simulink model "Enc"  (R2022b)
settings: Solver=FixedStepDiscrete  StartTime=0.0  StopTime=10.0  FixedStep=0.1  RelTol=1e-3
undefined symbols (not defined in the file): ParamCfg_Avgcnt_u16, ParamCfg_Cosamp_u16, ParamCfg_Cosavg_u16, ParamCfg_Sinamp_u16, ParamCfg_Sinavg_u16
libraries: simulink x2, dspsrcs4 x1
settings Model: DataDictionary=MCU_Input_Sldd.sldd  Creator=ZYH  LastModifiedBy=ZYH
settings OptimizationCC: DefaultParameterBehavior=Inlined  DefaultUnderspecifiedDataType=single  EnhancedBackFolding=on  PassReuseOutputArgsAs=Individual arguments  ZeroExternalMemoryAtStartup=off  ZeroInternalMemoryAtStartup=off  OptimizeBlockOrder=speed  DifferentSizesBufferReuse=on  OptimizationCustomize=off  EfficientTunableParamExpr=on
settings DebuggingCC: ParameterTunabilityLossMsg=error
settings SFSimCC: MATLABDynamicMemAlloc=off
settings RTWCC: Description=Embedded Coder  SystemTargetFile=ert.tlc  GenCodeOnly=on  TemplateMakefile=ert_default_tmf
settings CodeAppCC: IgnoreCustomStorageClasses=off  MaxIdLength=40  OperatorAnnotations=on  SimulinkDataObjDesc=on  SFDataObjDesc=on  SimulinkBlockComments=off
settings ERTTargetCC: TargetLangStandard=C99 (ISO)  GenerateSampleERTMain=on  InlinedParameterPlacement=NonHierarchical  ERTCustomFileTemplate=example_file_process.tlc

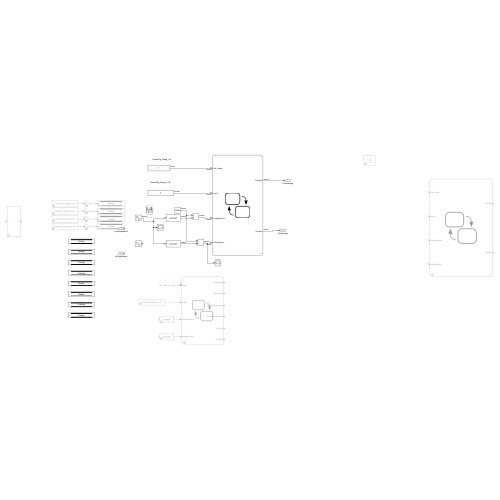
[thumbnail: Simulink's stored preview of the top-level diagram]
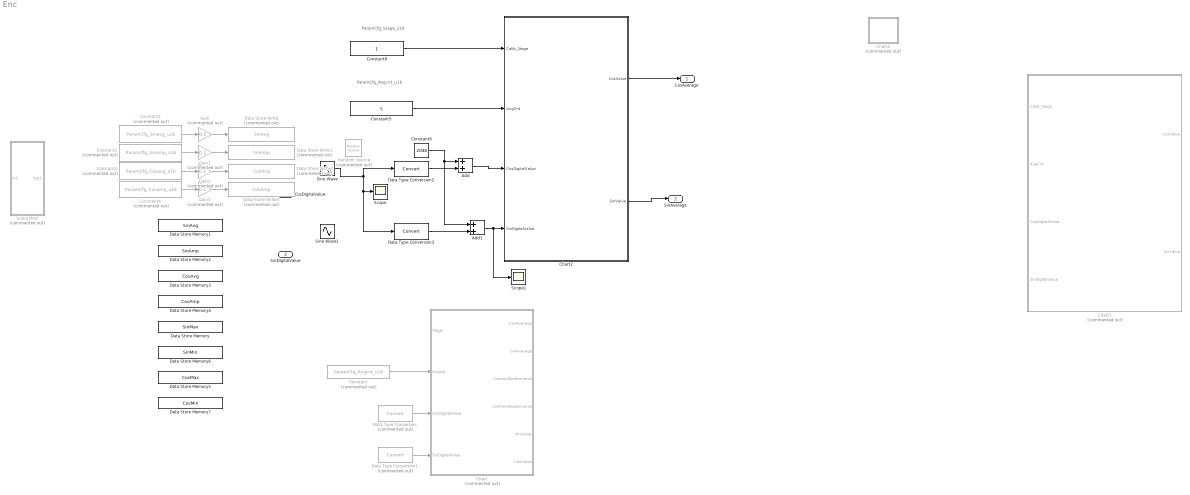
== system Enc ==
  note: ParamCfg_Stage_u16
  note: ParamCfg_Avgcnt_u16
  CosDigitalValue : Inport
  SinDigitalValue : Inport  Port=2
  Add : Sum
  Add1 : Sum
  Chart : Stateflow chart  Commented=on  TreatAsAtomicUnit=on
  Chart1 : Stateflow chart  Commented=on  TreatAsAtomicUnit=on
  Chart2 : Stateflow chart  TreatAsAtomicUnit=on
  Chart3 : Stateflow chart  Commented=on  TreatAsAtomicUnit=on
  Constant : Constant  Commented=on  Value=ParamCfg_Avgcnt_u16
  Constant1 : Constant  Commented=on  Value=ParamCfg_Sinavg_u16
  Constant2 : Constant  Commented=on  Value=ParamCfg_Sinamp_u16
  Constant3 : Constant  Commented=on  Value=ParamCfg_Cosavg_u16
  Constant4 : Constant  Commented=on  Value=ParamCfg_Cosamp_u16
  Constant5 : Constant  Value=5
  Constant6 : Constant  Value=2048
  Constant8 : Constant  OutDataTypeStr=uint16
  Data Store Memory : DataStoreMemory  DataStoreName=SinMax  WriteAfterWriteMsg=warning  InitialValue=2048  ShowAdditionalParam=off
  Data Store Memory1 : DataStoreMemory  DataStoreName=SinAvg  WriteAfterWriteMsg=warning  InitialValue=ParamCfg_Sinavg_u16  ShowAdditionalParam=off  OutDataTypeStr=uint16  StateMustResolveToSignalObject=on
  Data Store Memory2 : DataStoreMemory  DataStoreName=SinAmp  WriteAfterWriteMsg=warning  InitialValue=ParamCfg_Sinamp_u16  ShowAdditionalParam=off  OutDataTypeStr=uint16
  Data Store Memory3 : DataStoreMemory  DataStoreName=CosAvg  WriteAfterWriteMsg=warning  InitialValue=ParamCfg_Cosavg_u16  ShowAdditionalParam=off  OutDataTypeStr=uint16  StateMustResolveToSignalObject=on
  Data Store Memory4 : DataStoreMemory  DataStoreName=CosAmp  WriteAfterWriteMsg=warning  InitialValue=ParamCfg_Cosamp_u16  ShowAdditionalParam=off  OutDataTypeStr=uint16
  Data Store Memory5 : DataStoreMemory  DataStoreName=CosMax  WriteAfterWriteMsg=warning  InitialValue=2048  ShowAdditionalParam=off
  Data Store Memory6 : DataStoreMemory  DataStoreName=SinMin  WriteAfterWriteMsg=warning  InitialValue=2048  ShowAdditionalParam=off
  Data Store Memory7 : DataStoreMemory  DataStoreName=CosMin  WriteAfterWriteMsg=warning  InitialValue=2048  ShowAdditionalParam=off
  Data Store Write : DataStoreWrite  Commented=on  DataStoreName=SinAvg  IndexOptions=Index vector (dialog)  Indices=1  OutputSizes=1
  Data Store Write1 : DataStoreWrite  Commented=on  DataStoreName=SinAmp  IndexOptions=Index vector (dialog)  Indices=1  OutputSizes=1
  Data Store Write2 : DataStoreWrite  Commented=on  DataStoreName=CosAvg  IndexOptions=Index vector (dialog)  Indices=1  OutputSizes=1
  Data Store Write3 : DataStoreWrite  Commented=on  DataStoreName=CosAmp  IndexOptions=Index vector (dialog)  Indices=1  OutputSizes=1
  Data Type Conversion : DataTypeConversion  Commented=on  SaturateOnIntegerOverflow=off  RndMeth=Floor
  Data Type Conversion1 : DataTypeConversion  Commented=on  SaturateOnIntegerOverflow=off  RndMeth=Floor
  Data Type Conversion2 : DataTypeConversion  SaturateOnIntegerOverflow=off  RndMeth=Floor
  Data Type Conversion3 : DataTypeConversion  SaturateOnIntegerOverflow=off  RndMeth=Floor
  Gain{,1..3} (4 alike) : Gain  Commented=on  Gain=0.1  ParamDataTypeStr=single  OutDataTypeStr=single
  Random Source : dspsrcs4/Random Source  Commented=on  SrcType=Uniform  NormMethod=Ziggurat  CltLength=12  MinVal=1  MaxVal=10  MeanVal=0  VarVal=1  RepMode=Not repeatable  rawSeed=1  IsInherit=off  SampMode=Discrete  SampTime=1  SampFrame=1  DataType=Double  OutComplex=Real  OutputFrames=off
  Scope : Scope
  Scope1 : Scope
  Sine Wave : Sin  Amplitude=2  Phase=pi/2  SampleTime=0
  Sine Wave1 : Sin  Amplitude=0  SampleTime=0
  Subsystem : Subsystem  Commented=on
  CosAverage : Outport
  SinAverage : Outport  Port=2
  wires:
  ? -> Chart/1(Stage)
  Constant/1 -> Chart/2(Avgcnt)
  Data Type Conversion/1 -> Chart/3(CosDigitalValue)
  Data Type Conversion1/1 -> Chart/4(SinDigitalValue)
  Constant1/1 -> Gain/1
  Constant2/1 -> Gain1/1
  Gain/1 -> Data Store Write/1
  Gain1/1 -> Data Store Write1/1
  Constant3/1 -> Gain2/1
  Constant4/1 -> Gain3/1
  Gain2/1 -> Data Store Write2/1
  Gain3/1 -> Data Store Write3/1
  Sine Wave/1 -> Data Type Conversion2/1, Data Type Conversion3/1, Scope/1
  Chart2/1(CosValue) -> CosAverage/1
  Chart2/2(SinValue) -> SinAverage/1
  Constant8/1 -> Chart2/1(Calib_Stage)
  Constant5/1 -> Chart2/2(AvgCnt)
  Data Type Conversion2/1 -> Add/2
  Data Type Conversion3/1 -> Add1/2
  Add1/1 -> Scope1/1, Chart2/4(SinDigitalValue)
  Constant6/1 -> Add1/1, Add/1
  Add/1 -> Chart2/3(CosDigitalValue)

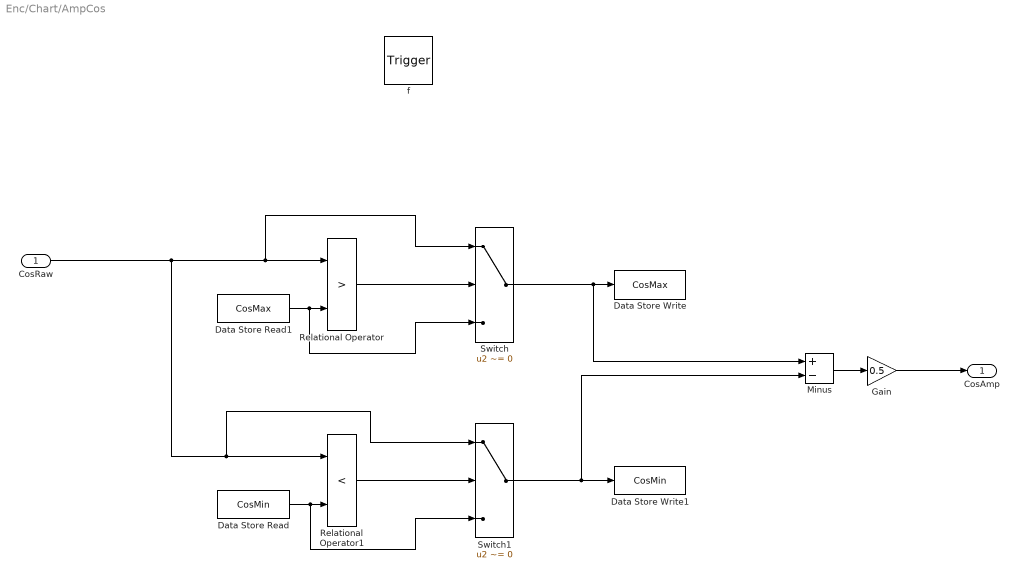
== system Enc/Chart/AmpCos ==
  CosRaw : Inport
  f : TriggerPort  TriggerType=function-call  VariantControl=(inherit)
      settings: CopyFcn=Stateflow.SLINSF.SimulinkMan.removeBlockPreDeleteFcn  PreDeleteFcn=Stateflow.SLINSF.SimulinkMan.unsafePredeleteFcn
  Data Store Read : DataStoreRead  DataStoreName=CosMin  IndexOptions=Index vector (dialog)  Indices=1  OutputSizes=1
  Data Store Read1 : DataStoreRead  DataStoreName=CosMax  IndexOptions=Index vector (dialog)  Indices=1  OutputSizes=1
  Data Store Write : DataStoreWrite  DataStoreName=CosMax  IndexOptions=Index vector (dialog)  Indices=1  OutputSizes=1
  Data Store Write1 : DataStoreWrite  DataStoreName=CosMin  IndexOptions=Index vector (dialog)  Indices=1  OutputSizes=1
  Gain : Gain  Gain=0.5
  Minus : Sum  Inputs=+-
  Relational Operator : RelationalOperator  Operator=>  OutDataTypeStr=boolean  RndMeth=Simplest  InputSameDT=off
  Relational Operator1 : RelationalOperator  Operator=<  OutDataTypeStr=boolean  RndMeth=Simplest  InputSameDT=off
  Switch : Switch  Criteria=u2 ~= 0  SaturateOnIntegerOverflow=off  InputSameDT=off
  Switch1 : Switch  Criteria=u2 ~= 0  SaturateOnIntegerOverflow=off  InputSameDT=off
  CosAmp : Outport
  wires:
  CosRaw/1 -> Switch1/1, Relational Operator1/1, Switch/1, Relational Operator/1
  Data Store Read1/1 -> Switch/3, Relational Operator/2
  Relational Operator/1 -> Switch/2
  Switch/1 -> Minus/1, Data Store Write/1
  Data Store Read/1 -> Switch1/3, Relational Operator1/2
  Relational Operator1/1 -> Switch1/2
  Switch1/1 -> Minus/2, Data Store Write1/1
  Minus/1 -> Gain/1
  Gain/1 -> CosAmp/1

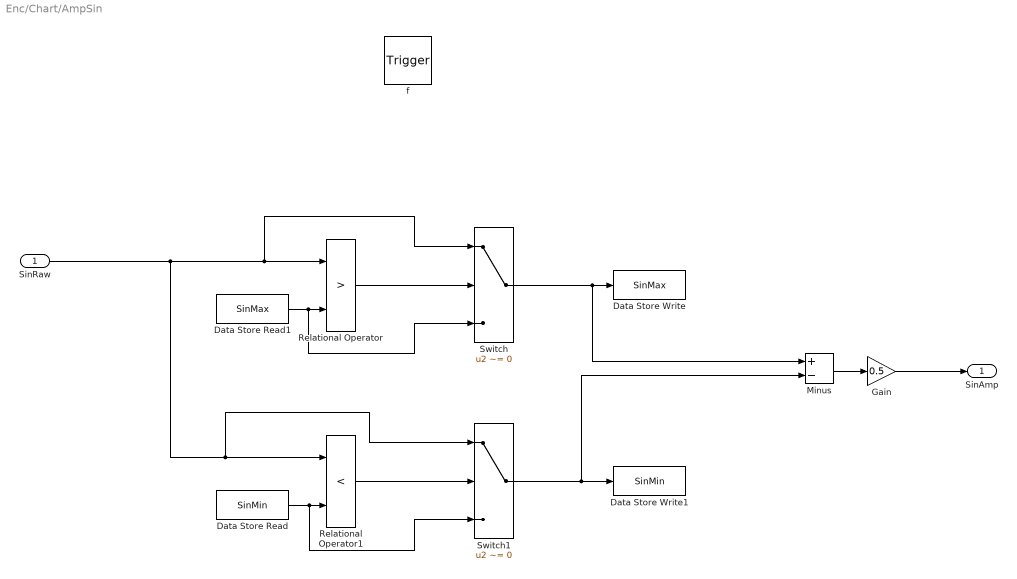
== system Enc/Chart/AmpSin ==
  SinRaw : Inport
  f : TriggerPort  TriggerType=function-call  VariantControl=(inherit)
      settings: CopyFcn=Stateflow.SLINSF.SimulinkMan.removeBlockPreDeleteFcn  PreDeleteFcn=Stateflow.SLINSF.SimulinkMan.unsafePredeleteFcn
  Data Store Read : DataStoreRead  DataStoreName=SinMin  IndexOptions=Index vector (dialog)  Indices=1  OutputSizes=1
  Data Store Read1 : DataStoreRead  DataStoreName=SinMax  IndexOptions=Index vector (dialog)  Indices=1  OutputSizes=1
  Data Store Write : DataStoreWrite  DataStoreName=SinMax  IndexOptions=Index vector (dialog)  Indices=1  OutputSizes=1
  Data Store Write1 : DataStoreWrite  DataStoreName=SinMin  IndexOptions=Index vector (dialog)  Indices=1  OutputSizes=1
  Gain : Gain  Gain=0.5
  Minus : Sum  Inputs=+-
  Relational Operator : RelationalOperator  Operator=>  OutDataTypeStr=boolean  RndMeth=Simplest  InputSameDT=off
  Relational Operator1 : RelationalOperator  Operator=<  OutDataTypeStr=boolean  RndMeth=Simplest  InputSameDT=off
  Switch : Switch  Criteria=u2 ~= 0  SaturateOnIntegerOverflow=off  InputSameDT=off
  Switch1 : Switch  Criteria=u2 ~= 0  SaturateOnIntegerOverflow=off  InputSameDT=off
  SinAmp : Outport
  wires:
  SinRaw/1 -> Switch1/1, Relational Operator1/1, Switch/1, Relational Operator/1
  Data Store Read1/1 -> Switch/3, Relational Operator/2
  Relational Operator/1 -> Switch/2
  Switch/1 -> Minus/1, Data Store Write/1
  Data Store Read/1 -> Switch1/3, Relational Operator1/2
  Relational Operator1/1 -> Switch1/2
  Switch1/1 -> Minus/2, Data Store Write1/1
  Minus/1 -> Gain/1
  Gain/1 -> SinAmp/1

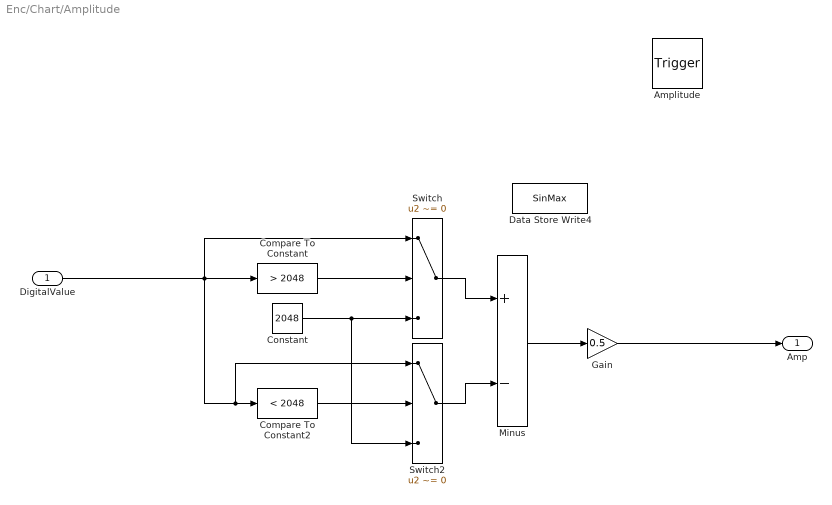
== system Enc/Chart/Amplitude ==
  DigitalValue : Inport  OutMin=0  OutMax=65535  OutDataTypeStr=uint16  PortDimensions=1
  Amplitude : TriggerPort  TriggerType=function-call  VariantControl=(inherit)
      settings: CopyFcn=Stateflow.SLINSF.SimulinkMan.removeBlockPreDeleteFcn  PreDeleteFcn=Stateflow.SLINSF.SimulinkMan.unsafePredeleteFcn
  Compare To Constant : simulink/Logic and Bit Operations/Compare To Constant  relop=>  const=2048  OutDataTypeStr=boolean
  Compare To Constant2 : simulink/Logic and Bit Operations/Compare To Constant  relop=<  const=2048  OutDataTypeStr=boolean
  Constant : Constant  Value=2048  OutDataTypeStr=uint16
  Data Store Write4 : DataStoreWrite  DataStoreName=SinMax  IndexOptions=Index vector (dialog)  Indices=1  OutputSizes=1
  Gain : Gain  Gain=0.5  OutDataTypeStr=single
  Minus : Sum  Inputs=+-
  Switch : Switch  Criteria=u2 ~= 0  SaturateOnIntegerOverflow=off  InputSameDT=off
  Switch2 : Switch  Criteria=u2 ~= 0  SaturateOnIntegerOverflow=off  InputSameDT=off
  Amp : Outport  PortDimensions=1
  wires:
  Compare To Constant/1 -> Switch/2
  Gain/1 -> Amp/1
  Compare To Constant2/1 -> Switch2/2
  Switch/1 -> Minus/1
  Switch2/1 -> Minus/2
  Constant/1 -> Switch2/3, Switch/3
  DigitalValue/1 -> Switch2/1, Compare To Constant2/1, Switch/1, Compare To Constant/1
  Minus/1 -> Gain/1

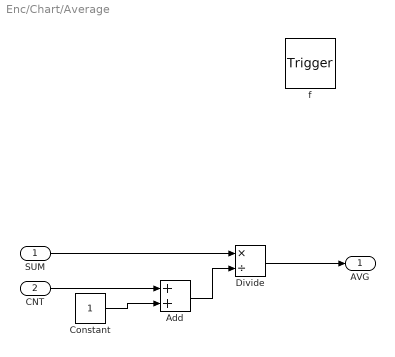
== system Enc/Chart/Average ==
  SUM : Inport  OutDataTypeStr=uint32  PortDimensions=1
  CNT : Inport  Port=2  OutDataTypeStr=uint16  PortDimensions=1
  f : TriggerPort  TriggerType=function-call  VariantControl=(inherit)
      settings: CopyFcn=Stateflow.SLINSF.SimulinkMan.removeBlockPreDeleteFcn  PreDeleteFcn=Stateflow.SLINSF.SimulinkMan.unsafePredeleteFcn
  Add : Sum  OutDataTypeStr=uint16
  Constant : Constant  OutDataTypeStr=uint16
  Divide : Product  Inputs=*/  OutDataTypeStr=single
  AVG : Outport  PortDimensions=1
  wires:
  CNT/1 -> Add/1
  Constant/1 -> Add/2
  SUM/1 -> Divide/1
  Add/1 -> Divide/2
  Divide/1 -> AVG/1

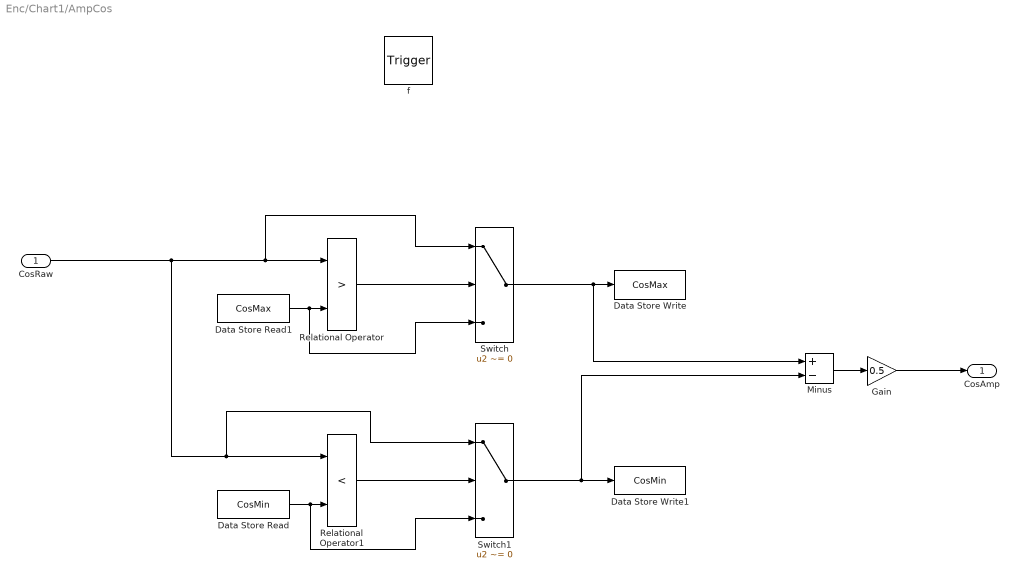
== system Enc/Chart1/AmpCos ==
  CosRaw : Inport  OutDataTypeStr=uint16  PortDimensions=1
  f : TriggerPort  TriggerType=function-call  VariantControl=(inherit)
      settings: CopyFcn=Stateflow.SLINSF.SimulinkMan.removeBlockPreDeleteFcn  PreDeleteFcn=Stateflow.SLINSF.SimulinkMan.unsafePredeleteFcn
  Data Store Read : DataStoreRead  DataStoreName=CosMin  IndexOptions=Index vector (dialog)  Indices=1  OutputSizes=1
  Data Store Read1 : DataStoreRead  DataStoreName=CosMax  IndexOptions=Index vector (dialog)  Indices=1  OutputSizes=1
  Data Store Write : DataStoreWrite  DataStoreName=CosMax  IndexOptions=Index vector (dialog)  Indices=1  OutputSizes=1
  Data Store Write1 : DataStoreWrite  DataStoreName=CosMin  IndexOptions=Index vector (dialog)  Indices=1  OutputSizes=1
  Gain : Gain  Gain=0.5  ParamDataTypeStr=single  OutDataTypeStr=single
  Minus : Sum  Inputs=+-
  Relational Operator : RelationalOperator  Operator=>  OutDataTypeStr=boolean  RndMeth=Simplest  InputSameDT=off
  Relational Operator1 : RelationalOperator  Operator=<  OutDataTypeStr=boolean  RndMeth=Simplest  InputSameDT=off
  Switch : Switch  Criteria=u2 ~= 0  SaturateOnIntegerOverflow=off  InputSameDT=off
  Switch1 : Switch  Criteria=u2 ~= 0  SaturateOnIntegerOverflow=off  InputSameDT=off
  CosAmp : Outport  OutDataTypeStr=single
  wires:
  CosRaw/1 -> Switch1/1, Relational Operator1/1, Switch/1, Relational Operator/1
  Data Store Read1/1 -> Switch/3, Relational Operator/2
  Relational Operator/1 -> Switch/2
  Switch/1 -> Minus/1, Data Store Write/1
  Data Store Read/1 -> Switch1/3, Relational Operator1/2
  Relational Operator1/1 -> Switch1/2
  Switch1/1 -> Minus/2, Data Store Write1/1
  Minus/1 -> Gain/1
  Gain/1 -> CosAmp/1

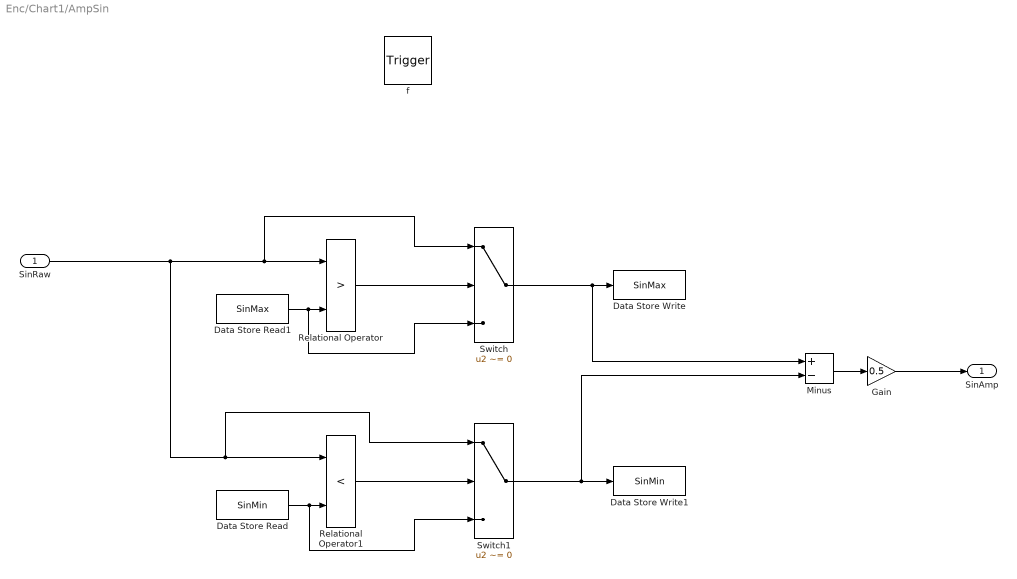
== system Enc/Chart1/AmpSin ==
  SinRaw : Inport  OutDataTypeStr=uint16  PortDimensions=1
  f : TriggerPort  TriggerType=function-call  VariantControl=(inherit)
      settings: CopyFcn=Stateflow.SLINSF.SimulinkMan.removeBlockPreDeleteFcn  PreDeleteFcn=Stateflow.SLINSF.SimulinkMan.unsafePredeleteFcn
  Data Store Read : DataStoreRead  DataStoreName=SinMin  IndexOptions=Index vector (dialog)  Indices=1  OutputSizes=1
  Data Store Read1 : DataStoreRead  DataStoreName=SinMax  IndexOptions=Index vector (dialog)  Indices=1  OutputSizes=1
  Data Store Write : DataStoreWrite  DataStoreName=SinMax  IndexOptions=Index vector (dialog)  Indices=1  OutputSizes=1
  Data Store Write1 : DataStoreWrite  DataStoreName=SinMin  IndexOptions=Index vector (dialog)  Indices=1  OutputSizes=1
  Gain : Gain  Gain=0.5  ParamDataTypeStr=single  OutDataTypeStr=single
  Minus : Sum  Inputs=+-
  Relational Operator : RelationalOperator  Operator=>  OutDataTypeStr=boolean  RndMeth=Simplest  InputSameDT=off
  Relational Operator1 : RelationalOperator  Operator=<  OutDataTypeStr=boolean  RndMeth=Simplest  InputSameDT=off
  Switch : Switch  Criteria=u2 ~= 0  SaturateOnIntegerOverflow=off  InputSameDT=off
  Switch1 : Switch  Criteria=u2 ~= 0  SaturateOnIntegerOverflow=off  InputSameDT=off
  SinAmp : Outport  OutDataTypeStr=single  PortDimensions=1
  wires:
  SinRaw/1 -> Switch1/1, Relational Operator1/1, Switch/1, Relational Operator/1
  Data Store Read1/1 -> Switch/3, Relational Operator/2
  Relational Operator/1 -> Switch/2
  Switch/1 -> Minus/1, Data Store Write/1
  Data Store Read/1 -> Switch1/3, Relational Operator1/2
  Relational Operator1/1 -> Switch1/2
  Switch1/1 -> Minus/2, Data Store Write1/1
  Minus/1 -> Gain/1
  Gain/1 -> SinAmp/1

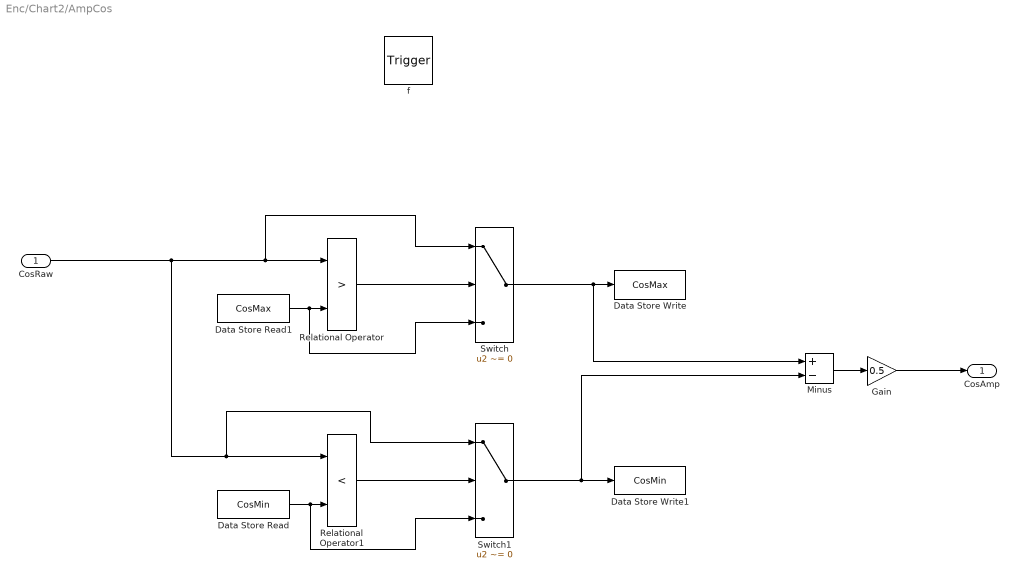
== system Enc/Chart2/AmpCos ==
  CosRaw : Inport  OutDataTypeStr=uint16  PortDimensions=1
  f : TriggerPort  TriggerType=function-call  VariantControl=(inherit)
      settings: CopyFcn=Stateflow.SLINSF.SimulinkMan.removeBlockPreDeleteFcn  PreDeleteFcn=Stateflow.SLINSF.SimulinkMan.unsafePredeleteFcn
  Data Store Read : DataStoreRead  DataStoreName=CosMin  IndexOptions=Index vector (dialog)  Indices=1  OutputSizes=1
  Data Store Read1 : DataStoreRead  DataStoreName=CosMax  IndexOptions=Index vector (dialog)  Indices=1  OutputSizes=1
  Data Store Write : DataStoreWrite  DataStoreName=CosMax  IndexOptions=Index vector (dialog)  Indices=1  OutputSizes=1
  Data Store Write1 : DataStoreWrite  DataStoreName=CosMin  IndexOptions=Index vector (dialog)  Indices=1  OutputSizes=1
  Gain : Gain  Gain=0.5  ParamDataTypeStr=single  OutDataTypeStr=single
  Minus : Sum  Inputs=+-
  Relational Operator : RelationalOperator  Operator=>  OutDataTypeStr=boolean  RndMeth=Simplest  InputSameDT=off
  Relational Operator1 : RelationalOperator  Operator=<  OutDataTypeStr=boolean  RndMeth=Simplest  InputSameDT=off
  Switch : Switch  Criteria=u2 ~= 0  SaturateOnIntegerOverflow=off  InputSameDT=off
  Switch1 : Switch  Criteria=u2 ~= 0  SaturateOnIntegerOverflow=off  InputSameDT=off
  CosAmp : Outport  OutDataTypeStr=single
  wires:
  CosRaw/1 -> Switch1/1, Relational Operator1/1, Switch/1, Relational Operator/1
  Data Store Read1/1 -> Switch/3, Relational Operator/2
  Relational Operator/1 -> Switch/2
  Switch/1 -> Minus/1, Data Store Write/1
  Data Store Read/1 -> Switch1/3, Relational Operator1/2
  Relational Operator1/1 -> Switch1/2
  Switch1/1 -> Minus/2, Data Store Write1/1
  Minus/1 -> Gain/1
  Gain/1 -> CosAmp/1

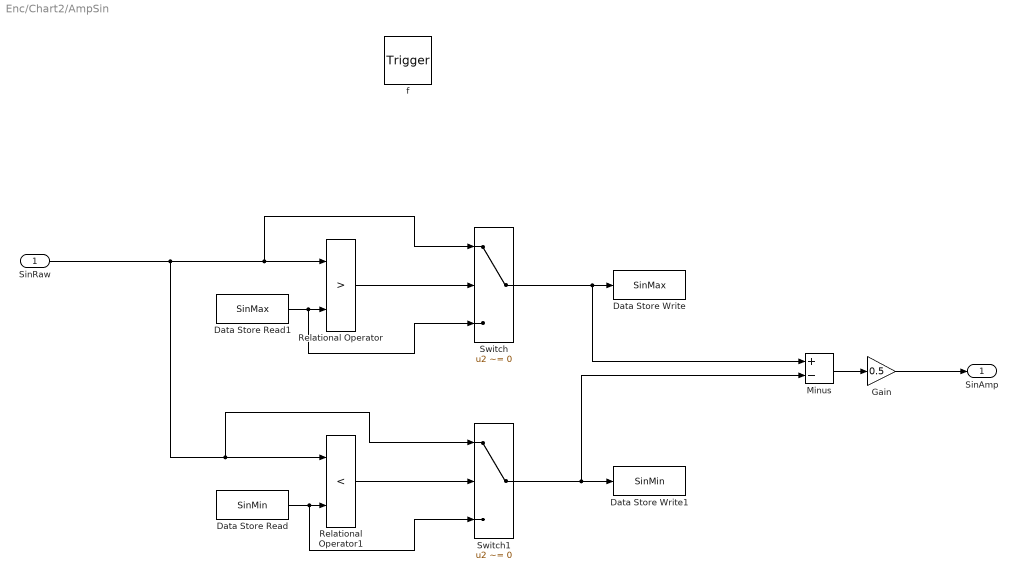
== system Enc/Chart2/AmpSin ==
  SinRaw : Inport  OutDataTypeStr=uint16  PortDimensions=1
  f : TriggerPort  TriggerType=function-call  VariantControl=(inherit)
      settings: CopyFcn=Stateflow.SLINSF.SimulinkMan.removeBlockPreDeleteFcn  PreDeleteFcn=Stateflow.SLINSF.SimulinkMan.unsafePredeleteFcn
  Data Store Read : DataStoreRead  DataStoreName=SinMin  IndexOptions=Index vector (dialog)  Indices=1  OutputSizes=1
  Data Store Read1 : DataStoreRead  DataStoreName=SinMax  IndexOptions=Index vector (dialog)  Indices=1  OutputSizes=1
  Data Store Write : DataStoreWrite  DataStoreName=SinMax  IndexOptions=Index vector (dialog)  Indices=1  OutputSizes=1
  Data Store Write1 : DataStoreWrite  DataStoreName=SinMin  IndexOptions=Index vector (dialog)  Indices=1  OutputSizes=1
  Gain : Gain  Gain=0.5  ParamDataTypeStr=single  OutDataTypeStr=single
  Minus : Sum  Inputs=+-
  Relational Operator : RelationalOperator  Operator=>  OutDataTypeStr=boolean  RndMeth=Simplest  InputSameDT=off
  Relational Operator1 : RelationalOperator  Operator=<  OutDataTypeStr=boolean  RndMeth=Simplest  InputSameDT=off
  Switch : Switch  Criteria=u2 ~= 0  SaturateOnIntegerOverflow=off  InputSameDT=off
  Switch1 : Switch  Criteria=u2 ~= 0  SaturateOnIntegerOverflow=off  InputSameDT=off
  SinAmp : Outport  OutDataTypeStr=single  PortDimensions=1
  wires:
  SinRaw/1 -> Switch1/1, Relational Operator1/1, Switch/1, Relational Operator/1
  Data Store Read1/1 -> Switch/3, Relational Operator/2
  Relational Operator/1 -> Switch/2
  Switch/1 -> Minus/1, Data Store Write/1
  Data Store Read/1 -> Switch1/3, Relational Operator1/2
  Relational Operator1/1 -> Switch1/2
  Switch1/1 -> Minus/2, Data Store Write1/1
  Minus/1 -> Gain/1
  Gain/1 -> SinAmp/1

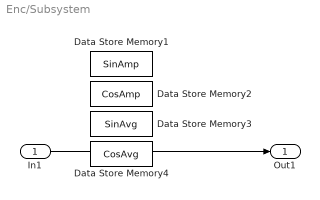
== system Enc/Subsystem ==
  In1 : Inport
  Data Store Memory1 : DataStoreMemory  DataStoreName=SinAmp  WriteAfterWriteMsg=warning  InitialValue=ParamCfg_Sinamp_u16  ShowAdditionalParam=off  OutDataTypeStr=single  StateMustResolveToSignalObject=on
  Data Store Memory2 : DataStoreMemory  DataStoreName=CosAmp  WriteAfterWriteMsg=warning  ShowAdditionalParam=off  OutDataTypeStr=single  StateMustResolveToSignalObject=on
  Data Store Memory3 : DataStoreMemory  DataStoreName=SinAvg  WriteAfterWriteMsg=warning  ShowAdditionalParam=off  OutDataTypeStr=single  StateMustResolveToSignalObject=on
  Data Store Memory4 : DataStoreMemory  DataStoreName=CosAvg  WriteAfterWriteMsg=warning  ShowAdditionalParam=off  OutDataTypeStr=single  StateMustResolveToSignalObject=on
  Out1 : Outport
  wires:
  In1/1 -> Out1/1

== stateflow chart Enc/Chart3 ==
  state A
  (default) -> (junction 3)
  (junction 3) -> A

== stateflow chart Enc/Chart1 ==
  state SinAmp = AmpSin(SinRaw) [function]
  state Normalize
    du:
    if(Cnt < AvgCnt)
    AmplitudeSin =AmpSin(SinDigitalValue);
    AmplitudeCos = AmpCos(CosDigitalValue);
    SinSum = SinSum + SinDigitalValue;
    CosSum = CosSum + CosDigitalValue;
    Cnt = Cnt + 1;
    else
    %求均值
    SinAverage = SinSum/(Cnt+1);
    CosAverage = CosSum/(Cnt+1);
    %求幅值倒数
    InvAmpSin = 1/AmplitudeSin;
    InvAmpCos = 1/AmplitudeCos;
    %更新参数
    end
    end
  state Compensate
  state CosAmp = AmpCos(CosRaw) [function]
  note: NormlizeSinCos
      |
      | du:
      | if(Cnt < Avgcnt)
      |     SinAmplitude = AmpSin(SinDigitalValue);
      |     CosAmplitude = AmpCos(CosDigitalValue);
      |     Cnt = Cnt+1;
      |     SinSum = SinSum + uint32(SinDigitalValue);
      |     CosSum = CosSum+ uint32(CosDigitalValue);
      | else
      |     SinAverage = Average(SinSum,Cnt);%single(SinSum/(Cnt+1));
      |     CosAverage = Average(CosSum,Cnt);%single(CosSum/(Cnt+1));
      |
      |     SinAmplitudeInverse = 1/SinAmplitude;
      |     CosAmplitudeInverse = 1/CosAmplitude;
      |
      |     SinAvg = SinAverage*10;
      |     CosAvg = CosAverage*10;
      |     SinAmp = SinAmplitude*10;
      |     CosAmp = CosAmplitude*10;
      | end
      | ToCalibFinish = true;
      | end
  state Finish
    du:
  (default) -> (junction 7)
  (junction 7) -> Compensate [order 3] : [Calib_Stage == COMPENSATE]
  (junction 7) -> Normalize [order 1] : [Calib_Stage == NORMALIZE]
  (junction 7) -> Finish [order 2]
  Compensate -> Finish
  Normalize -> Finish
  Finish -> (junction 23) : {
      | SinValue =1;
      | CosValue = 1;
      | }
  data: SinRaw function_input uint16 size=1; SinAmp function_output single size=1; CosRaw function_input uint16 size=1; CosAmp function_output single; Calib_Stage input; NORMALIZE constant double; COMPENSATE constant double; CosValue output; SinValue output; AvgCnt input; Cnt local; CosDigitalValue input; SinDigitalValue input; AmplitudeSin local single =single(0); AmplitudeCos local single =single(0); CosSum local s; SinSum local; CosAverage local; SinAverage local; InvAmpCos local; InvAmpSin local

== stateflow chart Enc/Chart2 ==
  note: Normalize
      |
      | du:
      | if(Cnt < AvgCnt)
      |     AmplitudeSin =AmpSin(SinDigitalValue);
      |     AmplitudeCos = AmpCos(CosDigitalValue);
      |     SinSum = SinSum + SinDigitalValue;
      |     CosSum = CosSum + CosDigitalValue;
      |     Cnt = Cnt + 1;
      | else
      |     %求均值
      |     SinAverage = SinSum/(Cnt+1);
      |     CosAverage = CosSum/(Cnt+1);
      |
      |     %求幅值倒数
      |     InvAmpSin = 1/AmplitudeSin;
      |     InvAmpCos = 1/AmplitudeCos;
      |
      |     %更新参数
      |
      | end
      | end
  note: Normalize
      |
      | du:
      | if(Cnt < AvgCnt)
      |     AmplitudeSin =AmpSin(SinDigitalValue);
      |     AmplitudeCos = AmpCos(CosDigitalValue);
      |     SinSum = SinSum + SinDigitalValue;
      |     CosSum = CosSum + CosDigitalValue;
      |     Cnt = Cnt + 1;
      | else
      |     %求均值
      |     SinAverage = SinSum/(Cnt+1);
      |     CosAverage = CosSum/(Cnt+1);
      |
      |     %求幅值倒数
      |     InvAmpSin = 1/AmplitudeSin;
      |     InvAmpCos = 1/AmplitudeCos;
      |
      |     %更新参数
      |
      | end
      | end
  state SinAmp = AmpSin(SinRaw) [function]
  state Normalize
    state A
      SinAmplitude =AmpSin(SinDigitalValue);
      CosAmplitude = AmpCos(CosDigitalValue);
      SinSum = SinSum + SinDigitalValue;
      CosSum = CosSum + CosDigitalValue;
      Cnt = Cnt+1;
    state B
      %求均值
      SinAverage = SinSum/(Cnt);
      CosAverage = CosSum/(Cnt);
      %求幅值倒数
      SinAmplitudeInverse = 1/SinAmplitude;
      CosAmplitudeInverse = 1/CosAmplitude;
      %更新参数
      SinAvg = SinAverage*10;
      CosAvg = CosAverage *10;
      SinAmp = SinAmplitude *10;
      CosAmp = CosAmplitude *10;
      %状态跳转
      ToFinish = 1
    (default) -> A
    (default) -> (junction 42) [commented out]
    (junction 42) -> ? [commented out] : [Cnt <AvgCnt]
        | {
        |     SinAmplitude =AmpSin(SinDigitalValue);
        |     CosAmplitude = AmpCos(CosDigitalValue);
        |     SinSum = SinSum + SinDigitalValue;
        |     CosSum = CosSum + CosDigitalValue;
        |     Cnt = Cnt + 1;
        | }
    (junction 42) -> ? [commented out] : {
        |     %求均值
        |     SinAverage = SinSum/(Cnt+1);
        |     CosAverage = CosSum/(Cnt+1);
        |
        |     %求幅值倒数
        |     SinAmplitudeInverse = 1/SinAmplitude;
        |     CosAmplitudeInverse = 1/CosAmplitude;
        |
        | %更新参数
        | SinAvg = SinAverage*10;
        | CosAvg = CosAverage *10;
        | SinAmp = SinAmplitude *10;
        | CosAmp = CosAmplitude *10;
        |
        | %状态跳转
        | ToFinish = 1
        | }
    A -> B : [Cnt > AvgCnt]
  state Compensate
  state CosAmp = AmpCos(CosRaw) [function]
  state Finish
    SinSum = 0;
    CosSum= 0;
    Cnt = 0;
    SinValue =(SinDigitalValue-SinAvg)*SinAmplitudeInverse;
    CosValue = (CosDigitalValue-CosAvg)*CosAmplitudeInverse;
  (default) -> (junction 7)
  (junction 7) -> Compensate [order 2] : [Calib_Stage == COMPENSATE]
  (junction 7) -> Normalize [order 1] : [Calib_Stage == NORMALIZE]
  (junction 7) -> Finish [order 3]
  Normalize -> Finish : [ToFinish == 1]
  Finish -> (junction 9) [commented out] : {
      | SinValue =(SinDigitalValue-SinAvg)*SinAmplitudeInverse;
      | CosValue = (CosDigitalValue-CosAvg)*CosAmplitudeInverse;
      | }
  data: SinRaw function_input uint16 size=1; SinAmp function_output single size=1; CosRaw function_input uint16 size=1; CosAmp function_output single; Calib_Stage input; AvgCnt input; CosDigitalValue input; SinDigitalValue input; CosValue output double; SinValue output double; Cnt local uint16 =0; CosSum local double; SinSum local double; COMPENSATE constant uint16 =2; NORMALIZE constant uint16 =1; SinAverage local double; CosAverage local double; CosAmplitudeInverse local double; SinAmplitudeInverse local double; CosAmplitude local double; SinAmplitude local double; CosAvg data_store_memory; SinAvg data_store_memory; SinAmp data_store_memory; CosAmp data_store_memory; ToFinish local uint8 =0

== stateflow chart Enc/Chart ==
  state CalibFinish
    du:
    Cnt = 0;
    SinSum = 0;
    CosSum = 0;
    ToCalibFinish = false;
    ToDown = true;
    end
  state SinAmp = AmpSin(SinRaw) [function]
  state IDLE
  state CosAmp = AmpCos(CosRaw) [function]
  state Amp = Amplitude(DigitalValue) [function] [commented out]
  state AVG = Average(SUM,CNT) [function] [commented out]
  state NormlizeSinCos
    du:
    if(Cnt < Avgcnt)
    SinAmplitude = AmpSin(SinDigitalValue);
    CosAmplitude = AmpCos(CosDigitalValue);
    Cnt = Cnt+1;
    SinSum = SinSum + uint32(SinDigitalValue);
    CosSum = CosSum+ uint32(CosDigitalValue);
    else
    SinAverage = Average(SinSum,Cnt);%single(SinSum/(Cnt+1));
    CosAverage = Average(CosSum,Cnt);%single(CosSum/(Cnt+1));
    SinAmplitudeInverse = 1/SinAmplitude;
    CosAmplitudeInverse = 1/CosAmplitude;
    SinAvg = SinAverage*10;
    CosAvg = CosAverage*10;
    SinAmp = SinAmplitude*10;
    CosAmp = CosAmplitude*10;
    end
    ToCalibFinish = true;
    end
  state CompPhaseShift
    SinSum = 1;
    CosSum = 1;
  state Down [commented out]
    du:
    SinValue = (single(SinDigitalValue)-SinAverage) *SinAmplitudeInverse;
    CosValue = (single(CosDigitalValue)-CosAverage)*CosAmplitudeInverse;
  state Up
    du:
    SinValue = (single(SinDigitalValue)-SinAvg) *SinAmplitudeInverse;
    CosValue = (single(CosDigitalValue)-CosAvg)*CosAmplitudeInverse;
  (default) -> (junction 82)
  (junction 82) -> CalibFinish [order 1] : [Stage == CalibFinish ]
  (junction 82) -> IDLE [order 2]
  IDLE -> (junction 18) : {
      | SinAmplitude = SinAmp;
      | CosAmplitude = CosAmp;
      | SinAverage = SinAvg;
      | CosAverage = CosAvg;
      | SinAmplitudeInverse = 1/SinAmplitude;
      | CosAmplitudeInverse = 1/CosAmplitude;
      | }
  (junction 18) -> (junction 21) [order 1] : [Stage == NormlizeSinCos]
  (junction 18) -> (junction 23) [order 2] : [Stage == CompPhaseShift]
  (junction 21) -> NormlizeSinCos
  (junction 23) -> CompPhaseShift
  NormlizeSinCos -> CalibFinish : [ToCalibFinish ==1]
  CalibFinish -> Up : [ToDown == true]
  data: SinRaw function_input; SinAmp function_output; CosRaw function_input; CosAmp function_output; DigitalValue function_input double size=1; Amp function_output double size=1; SUM function_input double size=1; AVG function_output double size=1; CNT function_input double size=1; Stage input uint16 size=1; NormlizeSinCos constant uint16 =1; CompPhaseShift constant uint16 =2; CosSum local uint32; Cnt local uint16; SinSum local uint32; Avgcnt input uint16 size=1; CosDigitalValue input uint16 size=1; SinDigitalValue input uint16 size=1; SinAmp data_store_memory; CosAmp data_store_memory; SinAvg data_store_memory; CosAvg data_store_memory; ToCalibFinish local boolean =false; CalibFinish constant uint16 =0; CosAverage output single size=1; SinAverage output single size=1; SinAmplitudeInverse output single size=1; CosAmplitudeInverse output single size=1; CosAmplitude local single; SinAmplitude local single; ToDown local boolean =false; SinValue output; CosValue output
